simulink model "eml_asteroids"  (R2015a)
settings: Solver=FixedStepDiscrete  StartTime=0.0  StopTime=inf  FixedStep=1  RelTol=1e-3
StopFcn:
  | obj = findobj( 'Tag', 'asteroids_fig');
  | if ~isempty(obj),
  |    close(obj);
  | end;
libraries: simulink x2
(part 2 of 2)

== matlab function eml_asteroids/Plot ==
  settings: fimath=|
      | fimath(...
      | 'RoundMode', 'floor',...
      | 'OverflowMode', 'wrap',...
      | 'ProductMode', 'KeepLSB', 'ProductWordLength', 32,...
      | 'SumMode', 'KeepLSB', 'SumWordLength', 32,...
      | 'CastBeforeSum', false)
  data: objs input; info input
function plot(objs,info)

coder.extrinsic('eml_asteroids_setup');
coder.extrinsic('set','gca','hold','text','sprintf');
coder.extrinsic('line','drawnow', 'num2str');
coder.extrinsic('eml_asteroids_handle_map');

persistent canvas;
persistent figs;
persistent info_fig;

persistent debris;

level = info(1);
ships = info(2);
score = info(3);

maxobjs = 64;
maxdebris = 128;

if isempty(figs)
    figs = zeros(1,maxobjs);
    debris = zeros(10,maxdebris);
end

objs1 = double(objs);

min_x = 0;
max_x = 400;
min_y = 0;
max_y = 400;

if isempty(canvas)
    canvas = eml_asteroids_setup; % external user defined M function
                                  % (we don't have support for function handles)
    set(canvas, 'Color', 'black');
    set(gca, 'Visible', 'off');
    set(gca, 'XLim', [min_x max_x]);
    set(gca, 'YLim', [min_y max_y]);
    hold('on');
end

if isempty(info_fig)
    info_fig = text(35,380,'LEVEL: 00   SHIPS: 00   SCORE: 0000000','Color','y','FontName','FixedWidth','FontSize',12);
end
str = sprintf('LEVEL: %02d   SHIPS: %02d   SCORE: %06d', ...
               double(level), double(ships), double(score));
set(info_fig,'String',str);

for i = 1:maxdebris
    cnt = debris(1,i);
    if cnt == 0
        continue
    end

    sfig = debris(10,i);
    
    cnt = cnt - 1;
    debris(1,i) = cnt;
    sl = debris(9,i);
    if cnt <= 0 || sl <= 0
        debris(1,i) = 0;
        sfigHandle = eml_asteroids_handle_map(sfig);
        set(sfigHandle, 'xdata', []);
        set(sfigHandle, 'ydata', []);
        continue;
    end

    sx = debris(2,i);
    sy = debris(3,i);
    sr = debris(4,i);
    sv = debris(5,i);
    sd = debris(6,i);
    sa = debris(7,i);
    sva = debris(8,i);
    cos_sa = cos(sa);
    sin_sa = sin(sa);
    cos_sd = cos(sd);
    sin_sd = sin(sd);
    sx1 = sx+cos_sd*sr+sl*cos_sa;
    sy1 = sy+sin_sd*sr+sl*sin_sa;
    sx2 = sx+cos_sd*sr-sl*cos_sa;
    sy2 = sy+sin_sd*sr-sl*sin_sa;
    if sfig == 0
        col = [qrand()*0.5+0.5 qrand()*0.5+0.5 qrand()*0.5+0.5];
        sfigHandle = line([sx1 sx2],[sy1 sy2],'Color',col);
        sfig = eml_asteroids_handle_map(-1, sfigHandle);
        debris(10,i) = sfig;
    else
        sfigHandle = eml_asteroids_handle_map(sfig);
        set(sfigHandle, 'xdata', [sx1 sx2]);
        set(sfigHandle, 'ydata', [sy1 sy2]);
    end
    sr = sr + sv;
    sa = sa + sva;
    debris(4,i) = sr;
    debris(7,i) = sa;
    sl = sl - 0.1;
    if sl < 0
        sl = 0;
    end
    debris(9,i) = sl;
    debris(8,i) = sva;
    sv = sv - 0.5;
    if sv < 0
        sv = 0;
    end
    debris(5,i) = sv;
end

for i = 1:maxobjs
    if objs1(1,i) == 0 % object deleted
        figobj = figs(i);
        if figobj ~= 0
            figobjHandle = eml_asteroids_handle_map(figobj);
            set(figobjHandle, 'xdata', []);
            set(figobjHandle, 'ydata', []);
        end
        continue
    end
    
    if objs1(1,i) == 4 && objs1(11,i) == 1 % explosion
        debris = new_explosion(debris,objs1(2,i),objs1(3,i),objs1(10,i));
        continue
    end

    [xs, ys, n] = get_object_data(objs1(:,i));

    %
    % Make polygon data closed
    %
    for k = n+1:length(xs)
        xs(k) = xs(1);
        ys(k) = ys(1);
    end

    figobj = figs(i);
    
    if figobj == 0,
        figobjHandle = line(xs, ys);
        figobj = eml_asteroids_handle_map(-1, figobjHandle);
        figs(i) = figobj;
        set(figobjHandle, 'Color', char(objs1(9,i)));
    else
        figobjHandle = eml_asteroids_handle_map(figobj);
        set(figobjHandle, 'xdata', xs);
        set(figobjHandle, 'ydata', ys);
        set(figobjHandle, 'Color', char(objs1(9,i)));
    end
end
drawnow;
%pause(1);

function y = qrand
    y = 0;
    y = rand();

function debris = new_explosion(debris,x,y,n)
    n0 = n;
    maxdebris = 128;
    q = 0;
    r = 0;
    for i = 1:maxdebris
        if debris(1,i) == 0
            q = rand();
            debris(1,i) = 50;
            debris(2,i) = x;
            debris(3,i) = y;
            r = rand();
            r = r*(n0/15) + (n0/15);
            debris(4,i) = r;
            q = rand();
            debris(5,i) = (n0/6)*q+(n0/10);
            q = rand();
            debris(6,i) = q*2*pi;
            q = rand();
            debris(7,i) = q*2*pi;
            q = rand();
            debris(8,i) = q*0.8 - 0.3;
            q = rand();
            debris(9,i) = q*2+3;
            n = n - 1;
            if n <= 0
                return
            end
        end
    end
%
% get_object_data
%
% Get point data given object
%
function [xs, ys, n] = get_object_data(obj)

id = obj(1);
x = obj(2);
y = obj(3);
arg = obj(4);
r = obj(10);

xs = zeros(1,16);
ys = zeros(1,16);
n = 0;
if id == 1,
    asteroid_x0 = double(asteroid_x());
    asteroid_y0 = double(asteroid_y());
    asteroid_r0 = double(asteroid_r());
    n = size(asteroid_x0,1);
    f = r/asteroid_r0;
    xs(1:n) = x + f * asteroid_x0 * cos(arg) - f * asteroid_y0 * sin(arg);
    ys(1:n) = y + f * asteroid_x0 * sin(arg) + f * asteroid_y0 * cos(arg);
elseif id == 2
    ship_x0 = double(ship_x());
    ship_y0 = double(ship_y());
    ship_r0 = double(ship_r());
    n = size(ship_x0,1);
    f = r/ship_r0;
    xs(1:n) = x + f * ship_x0 * cos(arg) - f * ship_y0 * sin(arg);
    ys(1:n) = y + f * ship_x0 * sin(arg) + f * ship_y0 * cos(arg);
elseif id == 3
    missile_x0 = double(missile_x());
    missile_y0 = double(missile_y());
    missile_r0 = double(missile_r());
    n = size(missile_x0,1);
    f = r/missile_r0;
    xs(1:n) = x + f * missile_x0 * cos(arg) - f * missile_y0 * sin(arg);
    ys(1:n) = y + f * missile_x0 * sin(arg) + f * missile_y0 * cos(arg);
elseif id == 5
    thrust_x0 = double(thrust_x());
    thrust_y0 = double(thrust_y());
    thrust_r0 = double(thrust_r());
    n = size(thrust_x0,1);
    f = r/thrust_r0;
    xs(1:n) = x + f * thrust_x0 * cos(arg) - f * thrust_y0 * sin(arg);
    ys(1:n) = y + f * thrust_x0 * sin(arg) + f * thrust_y0 * cos(arg);
end

%
% asteroid_x
% asteroid_y
%
% Returning asteroid x and y data
%

function r = asteroid_x
    my_fimath = fimath('MaxProductWordLength',32,'MaxSumWordLength',32,...
                       'ProductFractionLength',12,'ProductMode','SpecifyPrecision',...
                       'SumFractionLength',12,'SumMode','SpecifyPrecision');
    my_fitype = numerictype(1,32,12);
    r = fi([2 10 20 17 7 16 12 -7 -17 -21 -14 -8 -7]',my_fitype,my_fimath);

function r = asteroid_y
    my_fimath = fimath('MaxProductWordLength',32,'MaxSumWordLength',32,...
                       'ProductFractionLength',12,'ProductMode','SpecifyPrecision',...
                       'SumFractionLength',12,'SumMode','SpecifyPrecision');
    my_fitype = numerictype(1,32,12);
    r = fi([18 22 5 -4 -6 -10 -17 -19 -13 3 17 11 23]',my_fitype,my_fimath);

function r = asteroid_r
    my_fimath = fimath('MaxProductWordLength',32,'MaxSumWordLength',32,...
                       'ProductFractionLength',12,'ProductMode','SpecifyPrecision',...
                       'SumFractionLength',12,'SumMode','SpecifyPrecision');
    my_fitype = numerictype(1,32,12);
    r = fi(22,my_fitype,my_fimath);

function r = ship_x
    my_fimath = fimath('MaxProductWordLength',32,'MaxSumWordLength',32,...
                       'ProductFractionLength',12,'ProductMode','SpecifyPrecision',...
                       'SumFractionLength',12,'SumMode','SpecifyPrecision');
    my_fitype = numerictype(1,32,12);
    r = fi([-4,-2,-2,-4,8]',my_fitype,my_fimath);
    
function r = ship_y
    my_fimath = fimath('MaxProductWordLength',32,'MaxSumWordLength',32,...
                       'ProductFractionLength',12,'ProductMode','SpecifyPrecision',...
                       'SumFractionLength',12,'SumMode','SpecifyPrecision');
    my_fitype = numerictype(1,32,12);
    r = fi([4,1,-1,-4,0]',my_fitype,my_fimath);

function r = ship_r
    my_fimath = fimath('MaxProductWordLength',32,'MaxSumWordLength',32,...
                       'ProductFractionLength',12,'ProductMode','SpecifyPrecision',...
                       'SumFractionLength',12,'SumMode','SpecifyPrecision');
    my_fitype = numerictype(1,32,12);
    r = fi(10,my_fitype,my_fimath);    

function r = thrust_x
    my_fimath = fimath('MaxProductWordLength',32,'MaxSumWordLength',32,...
                       'ProductFractionLength',12,'ProductMode','SpecifyPrecision',...
                       'SumFractionLength',12,'SumMode','SpecifyPrecision');
    my_fitype = numerictype(1,32,12);
    r = fi([-2,-2,-6]',my_fitype,my_fimath);

function r = thrust_y
    my_fimath = fimath('MaxProductWordLength',32,'MaxSumWordLength',32,...
                       'ProductFractionLength',12,'ProductMode','SpecifyPrecision',...
                       'SumFractionLength',12,'SumMode','SpecifyPrecision');
    my_fitype = numerictype(1,32,12);
    r = fi([1,-1,0]',my_fitype,my_fimath);    

function r = thrust_r
    my_fimath = fimath('MaxProductWordLength',32,'MaxSumWordLength',32,...
                       'ProductFractionLength',12,'ProductMode','SpecifyPrecision',...
                       'SumFractionLength',12,'SumMode','SpecifyPrecision');
    my_fitype = numerictype(1,32,12);
    r = fi(6,my_fitype,my_fimath);        
    
function r = missile_x
    my_fimath = fimath('MaxProductWordLength',32,'MaxSumWordLength',32,...
                       'ProductFractionLength',12,'ProductMode','SpecifyPrecision',...
                       'SumFractionLength',12,'SumMode','SpecifyPrecision');
    my_fitype = numerictype(1,32,12);
    r = fi([-4,4,-4]',my_fitype,my_fimath);
    
function r = missile_y
    my_fimath = fimath('MaxProductWordLength',32,'MaxSumWordLength',32,...
                       'ProductFractionLength',12,'ProductMode','SpecifyPrecision',...
                       'SumFractionLength',12,'SumMode','SpecifyPrecision');
    my_fitype = numerictype(1,32,12);
    r = fi([-1,0,1]',my_fitype,my_fimath);

function r = missile_r
    my_fimath = fimath('MaxProductWordLength',32,'MaxSumWordLength',32,...
                       'ProductFractionLength',12,'ProductMode','SpecifyPrecision',...
                       'SumFractionLength',12,'SumMode','SpecifyPrecision');
    my_fitype = numerictype(1,32,12);
    r = fi(8,my_fitype,my_fimath);

function y = newtagindex
persistent cnt;
if isempty(cnt)
    cnt = 0;
end
cnt = cnt + 1;
y = cnt;

== matlab function eml_asteroids/Reset Ship Controls ==
  settings: fimath=|
      | fimath(...
      | 'RoundMode', 'floor',...
      | 'OverflowMode', 'wrap',...
      | 'ProductMode', 'KeepLSB', 'ProductWordLength', 32,...
      | 'SumMode', 'KeepLSB', 'SumWordLength', 32,...
      | 'CastBeforeSum', false)
  data: x input
function reset(x)

feval('eml_asteroids_reset_controls',x);
